simulink model "Model"  (R2021b)
settings: Solver=VariableStepAuto  StartTime=0.0  StopTime=200  RelTol=1e-3
values from neighbouring files (symbols this model uses):
  eta_init = [0,0,deg2rad(15)]    [parameters.m]
  nu_init = [35,0,0]    [parameters.m]
settings Model: Creator=jacob  LastModifiedBy=jacob

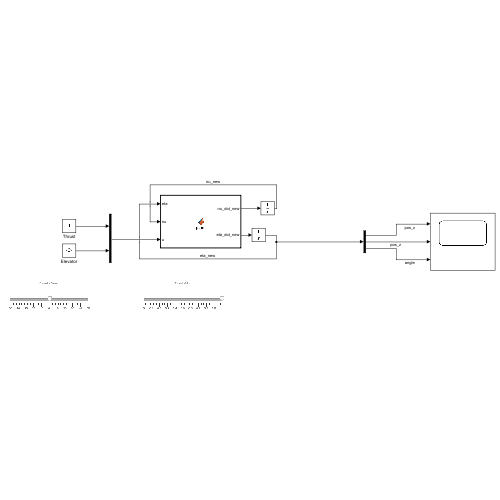
[thumbnail: Simulink's stored preview of the top-level diagram]
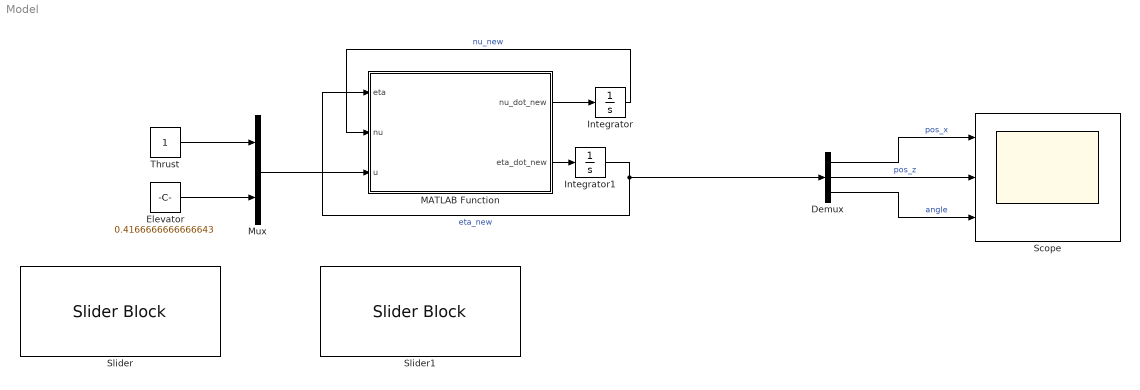
== system Model ==
  Demux : Demux  Outputs=3
  Elevator : Constant  Value=0.4166666666666643
  Integrator : Integrator  InitialCondition=nu_init
  Integrator1 : Integrator  InitialCondition=eta_init
  MATLAB Function : MATLAB Function  TreatAsAtomicUnit=on
  Mux : Mux  Inputs=2
  Scope : Scope  NumInputPorts=3
  Slider : SliderBlock  ScaleMin=-50  ScaleMax=50
  Slider1 : SliderBlock  ScaleMax=1
  Thrust : Constant
  wires:
  MATLAB Function/1(nu_dot_new) -> Integrator/1
  MATLAB Function/2(eta_dot_new) -> Integrator1/1
  Integrator/1 -> MATLAB Function/2(nu)  "nu_new"
  Integrator1/1 -> Demux/1, MATLAB Function/1(eta)  "eta_new"
  Thrust/1 -> Mux/1
  Mux/1 -> MATLAB Function/3(u)
  Elevator/1 -> Mux/2
  Demux/2 -> Scope/2  "pos_z"
  Demux/1 -> Scope/1  "pos_x"
  Demux/3 -> Scope/3  "angle"

== matlab function Model/MATLAB Function ==
  data: eta input; nu input; u input; nu_dot_new output size=[1,3]; eta_dot_new output size=[1,3]
function [nu_dot_new,eta_dot_new] = plant(eta,nu,u)

% ship parameters 
m = 13.5;          % mass (kg)
Jy = 1.135;         % pitch moment of inertia (kg m^3)
xg = 0;              % CG x-ccordinate (m)

%TODO: Add all params to a struct which is easier to pass to functions
% Aero parameters
rho = 1.2682; %air density 
alpha_0 = 0.4712; %rad
M = 50; %blending factor in aero coefficient calculation taken from beard&McLain appendix E

CL0 = 0.28; % Coefficient of lift at 0 pitch taken from beard&McLain appendix E
CL_alpha = 3.45; %Derivative of CL wrt. alpha taken from beard&McLain appendix E
CL_q = 0; %Derivative of CL wrt. q taken from beard&McLain appendix E
CL_deltaE = -0.36; %Derivative of CL wrt. deltaE taken from beard&McLain appendix E

CD0 = 0.03; % Coefficient of drag
CD_alpha = 0.3; %Derivative of CD wrt. alpha taken from beard&McLain appendix E
CD_q = 0; %Derivative of CD wrt. q taken from beard&McLain appendix E
CD_deltaE = 0; %Derivative of CD wrt. deltaE taken from beard&McLain appendix E
CD_p = 0.0437;

CM0 = -0.02338; % Aero moment coefficient
CM_alpha = -0.38; %Derivative of CM wrt. alpha taken from beard&McLain appendix E
CM_q = -3.6; %Derivative of CM wrt. q taken from beard&McLain appendix E
CM_deltaE = -0.5; %Derivative of CM wrt. deltaE taken from beard&McLain appendix E

S = 0.55;  %Wing area taken from beard&McLain appendix E
c = 0.18994;  %moment arm for wing taken from beard&McLain appendix E
b = 2.8956;%wingspan taken from beard&McLain appendix E
e = 0.9;

S_prop = 0.2027;%taken from beard&McLain appendix E
C_prop = 1; %just tuning here?
k_motor = 80; %taken from beard&McLain appendix E

deltaE = u(2);
deltaT = u(1);
theta = eta(3);
q = nu(3);
Va = sqrt(nu(1)*nu(1)+ nu(2)*nu(2));
alpha = atan2(nu(2),nu(1));%angle of attack


R_body_to_inertial = [cos(theta), sin(theta);
    -sin(theta), cos(theta)]; %Rotation matrix from body to inertial

R_inertial_to_body = R_body_to_inertial';


R_stab_to_body = [cos(alpha),-sin(alpha);
    sin(alpha), cos(alpha)]; %rotation from stability to body

%Compute gravity
FG = R_inertial_to_body*[0; m*9.81];

Fx_G = FG(1);
Fz_G = FG(2);

%Compute propeller thrust
Fx_thrust=0.5*rho*S_prop*C_prop*((k_motor*deltaT)*(k_motor*deltaT)-Va*Va);
fancyAero = 0;
if fancyAero

    [CL_ofAlpha, CD_ofAlpha] = computeAeroCoeffs(alpha, alpha_0, M, S, b, e, CL0, CD_p);


    CL = CL_ofAlpha + CL_q * 0.5*c*q/Va + CL_deltaE*deltaE;
    CD = CD_ofAlpha + CD_q * 0.5*c*q/Va + CD_deltaE*deltaE;

    F_lift = 0.5*rho*Va*Va*S*CL;
    F_drag = 0.5*rho*Va*Va*S*CD;

    CM = CM0 + CM_alpha * alpha;%+ CM_q*0.5*c*q/Va + CM_deltaE*deltaE;
    M_aero = 0.5*rho*Va*Va*S*c*CM/Jy;
else
    %Linear model
    %Compute areodynamic forces in stability frame
    CL = CL0 + CL_alpha*alpha + CL_q * 0.5*c*q/Va + CL_deltaE*deltaE;
    CD = CD0 + CD_alpha*alpha + CD_q * 0.5*c*q/Va + CD_deltaE*deltaE;
    CM = CM0 + CM_alpha*alpha + CM_q * 0.5*c*q/Va + CM_deltaE*deltaE;

    F_lift = 0.5 * rho * Va*Va * S * CL;
    F_drag = 0.5 * rho * Va*Va * S * CD;
    M_aero = (0.5 * rho * Va*Va * S * c * CM)/Jy;
end

F_aero = R_stab_to_body * [-F_drag;-F_lift]; %Transform to body frame

Fx_aero = F_aero(1);
Fz_aero = F_aero(2);

fx = Fx_G + Fx_aero - Fx_thrust;
fz = -Fz_G - Fz_aero;

CRB = nu(3)*[0, -1, 0;
    1, 0, 0;
    0, 0, 0];


F = [fx/m; fz/m; M_aero];


nu_dot = CRB * nu + F;

nu_mediate = nu(1:2);
eta_dot = [0;0;0];
eta_dot(1:2) = R_body_to_inertial * nu_mediate;
eta_dot(3) = nu(3);

eta_dot_new = eta_dot';
nu_dot_new = nu_dot';

end
